simulink model "VerticalFlight_TestModel"  (R2014a)
settings: Solver=ode3  StartTime=0.0  StopTime=25  FixedStep=0.01  MinStep=0.01  RelTol=1e-3
undefined symbols (not defined in the file or in its folder): dry_motor_weight, dry_rocket_weight, ground_launch_altitude, ground_pressure_ambient, ground_temperature_ambient, mass_flow_rate, wet_motor_weight
libraries: rocket_dynamic_data_library x3, rocket_isa_model_library x2, rocket_drag_library x2, rocket_vertical_flight_library x2
settings Model: Creator=scorpii  LastModifiedBy=scorpii
settings SolverCC: InitialStep=0.01
settings DataIOCC: LimitDataPoints=off
settings OptimizationCC: SimCompilerOptimization=off
settings DebuggingCC: ArtificialAlgebraicLoopMsg=error  MergeDetectMultiDrivingBlocksExec=error  FrameProcessingCompatibilityMsg=error
settings RTWCC: RTWCompilerOptimization=off

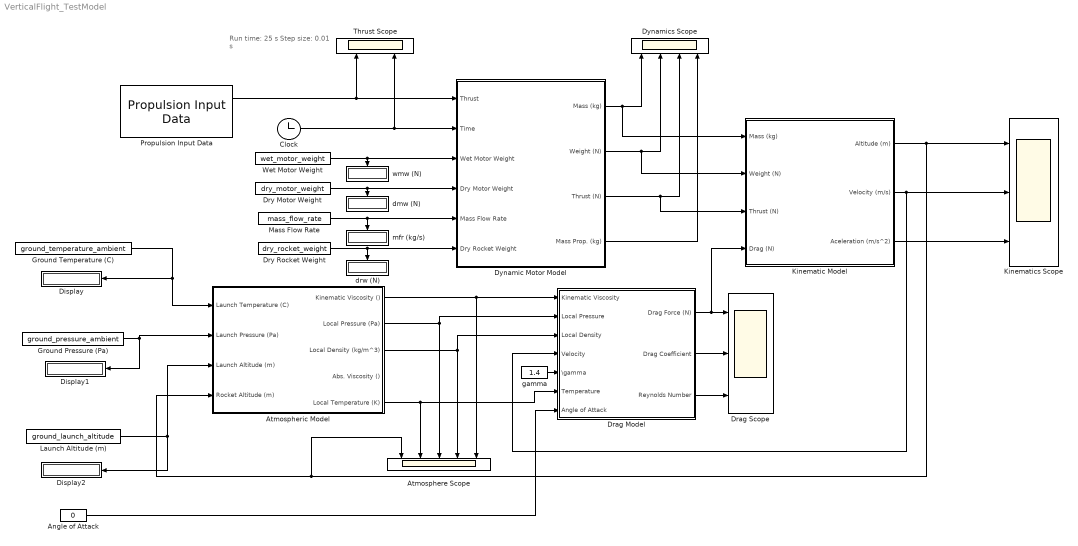
== system VerticalFlight_TestModel ==
  note: Run time: 25 s
      | Step size: 0.01 s
  Angle of Attack : Constant  Value=0
  Atmosphere Scope : Scope  NumInputPorts=5
      settings: YMin=-1~28.5~96258.8~11.1784~-1.12485e-07  YMax=1~31.5~106391~12.355~-1.01773e-07  SaveName=ScopeData4
  Atmospheric Model : Subsystem
  Clock : Clock
  Display : Display
  Display1 : Display
  Display2 : Display
  Drag Model : Subsystem
  Drag Scope : Scope  NumInputPorts=3
      settings: YMin=-5~-5~-5  YMax=5~5~5  SaveName=ScopeData3
  Dry Motor Weight : Constant  Value=dry_motor_weight
  Dry Rocket Weight : Constant  Value=dry_rocket_weight
  Dynamic Motor Model : Subsystem
  Dynamics Scope : Scope  NumInputPorts=4
      settings: YMin=126.243~1238.44~774.486~-5  YMax=139.531~1368.8~856.01~5
  Ground Pressure (Pa) : Constant  Value=ground_pressure_ambient
  Ground Temperature (C) : Constant  Value=ground_temperature_ambient
  Kinematic Model : Subsystem
  Kinematics Scope : Scope  NumInputPorts=3
      settings: YMin=0~-100~-80  YMax=600~150~110
  Launch Altitude (m) : Constant  Value=ground_launch_altitude
  Mass Flow Rate : Constant  Value=mass_flow_rate
  Propulsion Input Data : rocket_dynamic_data_library/Propulsion Input Data
  Thrust Scope : Scope  NumInputPorts=2
      settings: YMin=126.243~1238.44  YMax=139.531~1368.8  SaveName=ScopeData2
  Wet Motor Weight : Constant  Value=wet_motor_weight
  dmw (N) : Display
  drw (N) : Display
  gamma : Constant  Value=1.4
  mfr (kg/s) : Display
  wmw (N) : Display
  wires:
  Drag Model/1(Drag Force (N)) -> Drag Scope/1, Kinematic Model/4(Drag (N))
  Clock/1 -> Thrust Scope/2, Dynamic Motor Model/2(Time)
  Kinematic Model/1(Altitude (m)) -> Kinematics Scope/1, Atmospheric Model/4(Rocket Altitude (m)), Atmosphere Scope/1
  Kinematic Model/2(Velocity (m/s)) -> Kinematics Scope/2, Drag Model/4(Velocity)
  Kinematic Model/3(Aceleration (m/s^2)) -> Kinematics Scope/3
  Atmospheric Model/3(Local Density (kg/m^3)) -> Atmosphere Scope/4, Drag Model/3(Local Density)
  Atmospheric Model/2(Local Pressure (Pa)) -> Atmosphere Scope/3, Drag Model/2(Local Pressure)
  Atmospheric Model/1(Kinematic Viscosity ()) -> Atmosphere Scope/5, Drag Model/1(Kinematic Viscosity)
  Atmospheric Model/5(Local Temperature (K)) -> Atmosphere Scope/2, Drag Model/6(Temperature)
  Dynamic Motor Model/2(Weight (N)) -> Kinematic Model/2(Weight (N)), Dynamics Scope/2
  Dynamic Motor Model/1(Mass (kg)) -> Kinematic Model/1(Mass (kg)), Dynamics Scope/1
  Dynamic Motor Model/3(Thrust (N)) -> Kinematic Model/3(Thrust (N)), Dynamics Scope/3
  Propulsion Input Data/1 -> Dynamic Motor Model/1(Thrust), Thrust Scope/1
  Wet Motor Weight/1 -> Dynamic Motor Model/3(Wet Motor Weight), wmw (N)/1
  Dry Motor Weight/1 -> Dynamic Motor Model/4(Dry Motor Weight), dmw (N)/1
  Mass Flow Rate/1 -> Dynamic Motor Model/5(Mass Flow Rate), mfr (kg/s)/1
  Drag Model/2(Drag Coefficient) -> Drag Scope/2
  Drag Model/3(Reynolds Number) -> Drag Scope/3
  gamma/1 -> Drag Model/5(\gamma)
  Ground Temperature (C)/1 -> Display/1, Atmospheric Model/1(Launch Temperature (C))
  Ground Pressure (Pa)/1 -> Display1/1, Atmospheric Model/2(Launch Pressure (Pa))
  Launch Altitude (m)/1 -> Atmospheric Model/3(Launch Altitude (m)), Display2/1
  Dynamic Motor Model/4(Mass Prop. (kg)) -> Dynamics Scope/4
  Dry Rocket Weight/1 -> Dynamic Motor Model/6(Dry Rocket Weight), drw (N)/1
  Angle of Attack/1 -> Drag Model/7(Angle of Attack)

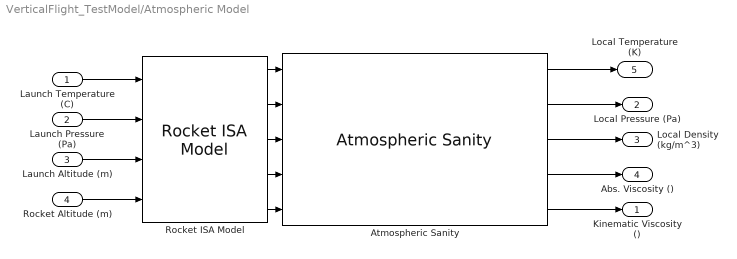
== system VerticalFlight_TestModel/Atmospheric Model ==
  Launch Temperature (C) : Inport
  Launch Pressure (Pa) : Inport  Port=2
  Launch Altitude (m) : Inport  Port=3
  Rocket Altitude (m) : Inport  Port=4
  Atmospheric Sanity : rocket_isa_model_library/Atmospheric Sanity
  Rocket ISA Model : rocket_isa_model_library/Rocket ISA Model
  Kinematic Viscosity () : Outport
  Local Pressure (Pa) : Outport  Port=2
  Local Density (kg/m^3) : Outport  Port=3
  Abs. Viscosity () : Outport  Port=4
  Local Temperature (K) : Outport  Port=5
  wires:
  Rocket ISA Model/5 -> Atmospheric Sanity/5
  Rocket ISA Model/2 -> Atmospheric Sanity/2
  Rocket ISA Model/3 -> Atmospheric Sanity/3
  Atmospheric Sanity/2 -> Local Pressure (Pa)/1
  Rocket ISA Model/4 -> Atmospheric Sanity/4
  Atmospheric Sanity/5 -> Kinematic Viscosity ()/1
  Atmospheric Sanity/1 -> Local Temperature (K)/1
  Atmospheric Sanity/3 -> Local Density (kg/m^3)/1
  Rocket ISA Model/1 -> Atmospheric Sanity/1
  Launch Temperature (C)/1 -> Rocket ISA Model/1
  Atmospheric Sanity/4 -> Abs. Viscosity ()/1
  Launch Pressure (Pa)/1 -> Rocket ISA Model/2
  Launch Altitude (m)/1 -> Rocket ISA Model/3
  Rocket Altitude (m)/1 -> Rocket ISA Model/4

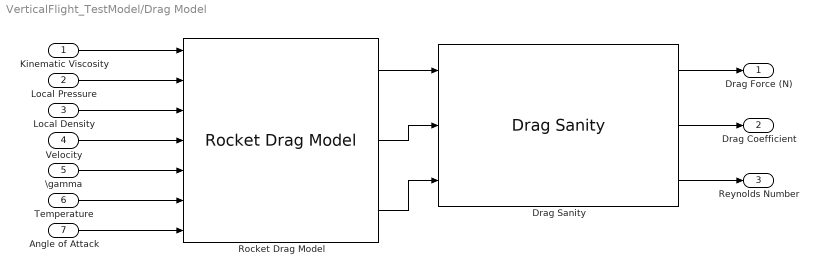
== system VerticalFlight_TestModel/Drag Model ==
  Kinematic Viscosity : Inport
  Local Pressure : Inport  Port=2
  Local Density : Inport  Port=3
  Velocity : Inport  Port=4
  \gamma : Inport  Port=5
  Temperature : Inport  Port=6
  Angle of Attack : Inport  Port=7
  Drag Sanity : rocket_drag_library/Drag Sanity
  Rocket Drag Model : rocket_drag_library/Rocket Drag Model
      link override Drag Force/BasicDrag: MATLABFcn=BasicDrag
      link override Rocket Drag Coefficient/Skin Friction Drag Coefficient/area_fin_frontal: Value=area_fin_frontal
      link override Skin Friction Drag Coefficient/Actual Reynolds Number/Reynolds Number (Actual): MATLABFcn=ReynoldsNumberActual
  Drag Force (N) : Outport
  Drag Coefficient : Outport  Port=2
  Reynolds Number : Outport  Port=3
  wires:
  Local Pressure/1 -> Rocket Drag Model/2
  Kinematic Viscosity/1 -> Rocket Drag Model/1
  Local Density/1 -> Rocket Drag Model/3
  Rocket Drag Model/3 -> Drag Sanity/3
  Rocket Drag Model/2 -> Drag Sanity/2
  Rocket Drag Model/1 -> Drag Sanity/1
  Drag Sanity/1 -> Drag Force (N)/1
  Drag Sanity/2 -> Drag Coefficient/1
  Drag Sanity/3 -> Reynolds Number/1
  Temperature/1 -> Rocket Drag Model/6
  Velocity/1 -> Rocket Drag Model/4
  \gamma/1 -> Rocket Drag Model/5
  Angle of Attack/1 -> Rocket Drag Model/7

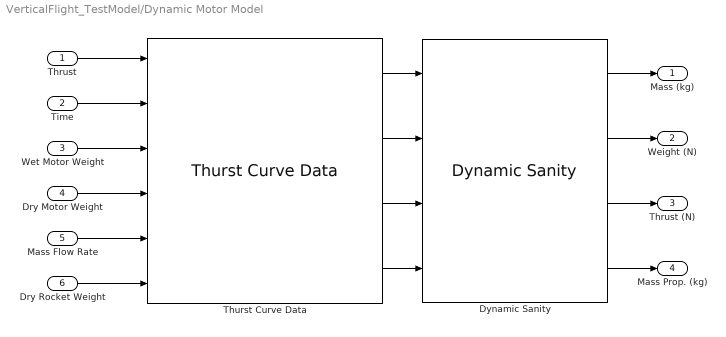
== system VerticalFlight_TestModel/Dynamic Motor Model ==
  Thrust : Inport
  Time : Inport  Port=2
  Wet Motor Weight : Inport  Port=3
  Dry Motor Weight : Inport  Port=4
  Mass Flow Rate : Inport  Port=5
  Dry Rocket Weight : Inport  Port=6
  Dynamic Sanity : rocket_dynamic_data_library/Dynamic Sanity
  Thurst Curve Data : rocket_dynamic_data_library/Thurst Curve Data
  Mass (kg) : Outport
  Weight (N) : Outport  Port=2
  Thrust (N) : Outport  Port=3
  Mass Prop. (kg) : Outport  Port=4
  wires:
  Time/1 -> Thurst Curve Data/2
  Dry Motor Weight/1 -> Thurst Curve Data/4
  Mass Flow Rate/1 -> Thurst Curve Data/5
  Dynamic Sanity/1 -> Mass (kg)/1
  Dynamic Sanity/3 -> Thrust (N)/1
  Wet Motor Weight/1 -> Thurst Curve Data/3
  Thrust/1 -> Thurst Curve Data/1
  Dynamic Sanity/2 -> Weight (N)/1
  Thurst Curve Data/1 -> Dynamic Sanity/1
  Thurst Curve Data/2 -> Dynamic Sanity/2
  Thurst Curve Data/3 -> Dynamic Sanity/3
  Thurst Curve Data/4 -> Dynamic Sanity/4
  Dynamic Sanity/4 -> Mass Prop. (kg)/1
  Dry Rocket Weight/1 -> Thurst Curve Data/6

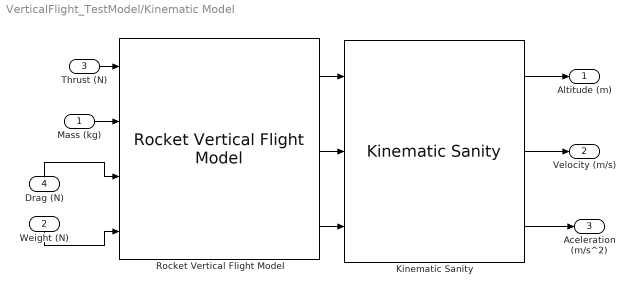
== system VerticalFlight_TestModel/Kinematic Model ==
  Mass (kg) : Inport
  Weight (N) : Inport  Port=2
  Thrust (N) : Inport  Port=3
  Drag (N) : Inport  Port=4
  Kinematic Sanity : rocket_vertical_flight_library/Kinematic Sanity
  Rocket Vertical Flight Model : rocket_vertical_flight_library/Rocket Vertical Flight Model
  Altitude (m) : Outport
  Velocity (m/s) : Outport  Port=2
  Aceleration (m/s^2) : Outport  Port=3
  wires:
  Rocket Vertical Flight Model/2 -> Kinematic Sanity/2
  Kinematic Sanity/2 -> Velocity (m/s)/1
  Rocket Vertical Flight Model/1 -> Kinematic Sanity/1
  Kinematic Sanity/3 -> Aceleration (m/s^2)/1
  Kinematic Sanity/1 -> Altitude (m)/1
  Rocket Vertical Flight Model/3 -> Kinematic Sanity/3
  Mass (kg)/1 -> Rocket Vertical Flight Model/2
  Weight (N)/1 -> Rocket Vertical Flight Model/4
  Thrust (N)/1 -> Rocket Vertical Flight Model/1
  Drag (N)/1 -> Rocket Vertical Flight Model/3
